simulink model "c960x4096_x14_7_r2013b_frb"  (R2013b)
(part 2 of 79)

      |     t = current_types(ctr);
      |     if (t < 0) || (t > 2),
      |         problem = t;
      |         ctr = numios + 1;
      |     end
      | end
      | if problem ~= 0,
      |     error('Type cannot be %i, must be 0, 1 or 2.', problem);
      | end
      mask Callback bin_pts:
      | swreg_maskcheck(gcb);
      | % blk = gcb;
      | % mode = get_param(blk, 'mode');
      | % current_bins = eval(get_param(blk, 'bin_pts'));
      | % if (strcmp(mode, 'one value') || strcmp(mode, 'fields of equal size')) && (length(current_bins) > 1),
      | %     error('Only one binary pt may be specified for this mode.');
      | % elseif strcmp(mode, 'fields of arbitrary size')
      | %     current_names = textscan(strtrim(strrep(strrep(get_param(blk, 'names'), ']', ''), '[', '')), '%s');
      | %     current_names = current_names{1};
      | %     numios = length(current_names);
      | %     if length(current_bins) ~= numios,
      | %         error('%d field names specified, but %d binary pts?', numios, length(current_bins));
      | %     end
      | % end
  trickler : Subsystem  mask{vec_len_bits=11}
      mask prompts: vec_len_bits "Vector Length (2^?)"
  trig : Subsystem  Tag=xps:sw_reg  AncestorBlock=xps_library/software register  mask(swreg){mode=one value, io_dir=From Processor, io_delay=0, sample_period=1, names=reg, bitwidths=32, arith_types=0, bin_pts=0, sim_port=on, show_format=off}
      mask prompts: io_dir "I/O direction"; io_delay "I/O delay"; sample_period "Sample period"; names "Name:"; bitwidths "Bitwidth:"; arith_types "Type (ufix=0, fix=1, bool=2):"; bin_pts "Binary pt:"; sim_port "Provide sim input/output?"; show_format "Print format string?"
      mask init:
      | swreg_init(gcb)
      settings: AttributesFormatString=1input
      mask TypeOptions mode: one value | fields of equal size | fields of arbitrary size
      mask Callback mode: swreg_cb(gcb);
      mask TypeOptions io_dir: To Processor | From Processor
      mask Callback io_dir:
      | mask_enables = get_param(gcb, 'MaskEnables');
      | mask_names = get_param(gcb, 'MaskNames');
      | if strcmp(get_param(gcb, 'io_dir'), 'To Processor'),
      |     mask_enables{ismember(mask_names, 'sample_period')} = 'off';
      | else
      |     mask_enables{ismember(mask_names, 'sample_period')} = 'on';
      | end
      | set_param(gcb, 'MaskEnables', mask_enables);
      mask Callback bitwidths:
      | swreg_maskcheck(gcb);
      | % blk = gcb;
      | % mode = get_param(blk, 'mode');
      | % current_widths = eval(get_param(blk, 'bitwidths'));
      | % if (strcmp(mode, 'one value') || strcmp(mode, 'fields of equal size')) && (length(current_widths) > 1),
      | %     error('Only one width may be specified for this mode.');
      | % elseif strcmp(mode, 'fields of arbitrary size')
      | %     current_names = textscan(strtrim(strrep(strrep(get_param(blk, 'names'), ']', ''), '[', '')), '%s');
      | %     current_names = current_names{1};
      | %     numios = length(current_names);
      | %     if length(current_widths) ~= numios,
      | %         error('%d field names specified, but %d widths?', numios, length(current_widths));
      | %     end
      | % end
      | % total_width = 0;
      | % for ctr = 1 : length(current_widths),
      | %     total_width = total_width + current_widths(ctr);
      | % end
      | % if total_width > 32,
      | %     error('Total width must be 32 or less, set to %d.', total_width);
      | % end
      mask Callback arith_types:
      | [numios, ~, ~, ~, current_types] = swreg_maskcheck(gcb);
      | % blk = gcb;
      | % mode = get_param(blk, 'mode');
      | % current_types = eval(get_param(blk, 'arith_types'));
      | % numios = length(current_types);
      | % if (strcmp(mode, 'one value') || strcmp(mode, 'fields of equal size')) && (length(current_types) > 1),
      | %     error('Only one type may be specified for this mode.');
      | % elseif strcmp(mode, 'fields of arbitrary size')
      | %     current_names = textscan(strtrim(strrep(strrep(get_param(blk, 'names'), ']', ''), '[', '')), '%s');
      | %     current_names = current_names{1};
      | %     numios = length(current_names);
      | %     if length(current_types) ~= numios,
      | %         error('%d field names specified, but %d types?', numios, length(current_types));
      | %     end
      | % end
      | problem = 0;
      | for ctr = 1 : numios,
      |     t = current_types(ctr);
      |     if (t < 0) || (t > 2),
      |         problem = t;
      |         ctr = numios + 1;
      |     end
      | end
      | if problem ~= 0,
      |     error('Type cannot be %i, must be 0, 1 or 2.', problem);
      | end
      mask Callback bin_pts:
      | swreg_maskcheck(gcb);
      | % blk = gcb;
      | % mode = get_param(blk, 'mode');
      | % current_bins = eval(get_param(blk, 'bin_pts'));
      | % if (strcmp(mode, 'one value') || strcmp(mode, 'fields of equal size')) && (length(current_bins) > 1),
      | %     error('Only one binary pt may be specified for this mode.');
      | % elseif strcmp(mode, 'fields of arbitrary size')
      | %     current_names = textscan(strtrim(strrep(strrep(get_param(blk, 'names'), ']', ''), '[', '')), '%s');
      | %     current_names = current_names{1};
      | %     numios = length(current_names);
      | %     if length(current_bins) ~= numios,
      | %         error('%d field names specified, but %d binary pts?', numios, length(current_bins));
      | %     end
      | % end
  tvg_cmult : Subsystem
  vacc : Subsystem
  wires:
  fftshift/1(in_reg) -> Delay16/1, Delay1/1
  Constant/1 -> fftshift/1(sim_1)
  scale_p0/1(in_reg) -> Delay2/1
  Constant29/1 -> scale_p0/1(sim_1)
  scale_p1/1(in_reg) -> Delay3/1
  Constant2/1 -> scale_p1/1(sim_1)
  ip_1/1(in_reg) -> Delay9/1
  Constant7/1 -> ip_1/1(sim_1)
  ip_2/1(in_reg) -> Delay10/1
  Constant8/1 -> ip_2/1(sim_1)
  ip_3/1(in_reg) -> Delay11/1
  Constant9/1 -> ip_3/1(sim_1)
  ip_4/1(in_reg) -> Delay12/1
  Constant10/1 -> ip_4/1(sim_1)
  ip_5/1(in_reg) -> Delay13/1
  Constant11/1 -> ip_5/1(sim_1)
  ip_6/1(in_reg) -> Delay14/1
  Constant12/1 -> ip_6/1(sim_1)
  ip_7/1(in_reg) -> Delay15/1
  Constant13/1 -> ip_7/1(sim_1)
  Constant15/1 -> pt_1/1(sim_1)
  Constant16/1 -> pt_2/1(sim_1)
  Constant17/1 -> pt_3/1(sim_1)
  Constant18/1 -> pt_4/1(sim_1)
  Constant19/1 -> pt_5/1(sim_1)
  Constant20/1 -> pt_6/1(sim_1)
  Constant21/1 -> pt_7/1(sim_1)
  arm/1(in_reg) -> Slice13/1
  [ADC_SYNC] -> Logical/1
  [P0_FFT_SYNC] -> leds/1(FFT_SYNC)
  [ADC_SYNC] -> leds/2(1PPS)
  Constant5/1 -> n_chan/1(sim_1)
  [TXOF] -> gbe_overflow/1(out_reg)
  Slice2/1 -> Delay4/1
  Register14/1 -> Register13/1
  Register28/1 -> Register27/1
  Register30/1 -> Register29/1
  Constant23/1 -> trig/1(sim_1)
  trig/1(in_reg) -> Slice4/1
  Constant27/1 -> adcsnap0/2(we)
  Constant26/1 -> adcsnap1/2(we)
  [trig] -> adcsnap0/3(trig)
  [trig] -> adcsnap1/3(trig)
  Register49/1 -> Register48/1
  Constant25/1 -> timesel/1(sim_1)
  timesel/1(in_reg) -> Convert16/1
  Convert16/1 -> Delay6/1
  Xilinx14_7/1 -> plat_bd/1(out_reg)
  p0_scale/7(S5_out) -> [P0_S5]
  p0_scale/5(S3_out) -> [P0_S3]
  p0_scale/3(S1_out) -> [P0_S1]
  p0_scale/9(S7_out) -> [P0_S7]
  p0_scale/4(S2_out) -> [P0_S2]
  p0_scale/6(S4_out) -> [P0_S4]
  p0_scale/8(S6_out) -> [P0_S6]
  p0_scale/2(SO_out) -> [P0_S0]
  p1_scale/2(SO_out) -> [P1_S0]
  p1_scale/7(S5_out) -> [P1_S5]
  p1_scale/9(S7_out) -> [P1_S7]
  p1_scale/6(S4_out) -> [P1_S4]
  p1_scale/3(S1_out) -> [P1_S1]
  p1_scale/4(S2_out) -> [P1_S2]
  p1_scale/5(S3_out) -> [P1_S3]
  p1_scale/8(S6_out) -> [P1_S6]
  [P0_S2] -> merge_pol/4(P0_S2)
  [P1_S6] -> merge_pol/16(P1_S6)
  [P0_S5] -> merge_pol/7(P0_S5)
  [P1_S5] -> merge_pol/15(P1_S5)
  [P1_S7] -> merge_pol/17(P1_S7)
  [P0_S4] -> merge_pol/6(P0_S4)
  [P0_S3] -> merge_pol/5(P0_S3)
  [P1_S3] -> merge_pol/13(P1_S3)
  [P1_S1] -> merge_pol/11(P1_S1)
  [P0_S7] -> merge_pol/9(P0_S7)
  [P0_S0] -> merge_pol/2(P0_S0)
  [P0_S1] -> merge_pol/3(P0_S1)
  [P1_S4] -> merge_pol/14(P1_S4)
  [P1_S0] -> merge_pol/10(P1_S0)
  [P0_S6] -> merge_pol/8(P0_S6)
  [P1_S2] -> merge_pol/12(P1_S2)
  [MDB1] -> ds_to_tgbe/2(DIN1)
  [MDB2] -> ds_to_tgbe/3(DIN2)
  [MDB3] -> ds_to_tgbe/4(DIN3)
  [MSYNC1] -> ds_to_tgbe/5(MSYNC)
  [SYNC] -> ds_to_tgbe/6(SYNCIN)
  [NCHAN] -> ds_to_tgbe/7(NCHAN)
  ds_to_tgbe/11(STB_3) -> [STB_3]
  ds_to_tgbe/19(DOUT_6) -> [DOUT_6]
  ds_to_tgbe/21(EOF_6) -> [EOF_6]
  ds_to_tgbe/18(EOF_5) -> [EOF_5]
  ds_to_tgbe/24(EOF_7) -> [EOF_7]
  ds_to_tgbe/22(DOUT_7) -> [DOUT_7]
  ds_to_tgbe/5(STB_1) -> [STB_1]
  ds_to_tgbe/17(STB_5) -> [STB_5]
  ds_to_tgbe/16(DOUT_5) -> [DOUT_5]
  ds_to_tgbe/3(EOF_0) -> [EOF_0]
  ds_to_tgbe/15(EOF_4) -> [EOF_4]
  ds_to_tgbe/14(STB_4) -> [STB_4]
  ds_to_tgbe/9(EOF_2) -> [EOF_2]
  ds_to_tgbe/10(DOUT_3) -> [DOUT_3]
  ds_to_tgbe/20(STB_6) -> [STB_6]
  ds_to_tgbe/23(STB_7) -> [STB_7]
  ds_to_tgbe/2(STB_0) -> [STB_0]
  ds_to_tgbe/12(EOF_3) -> [EOF_3]
  ds_to_tgbe/4(DOUT_1) -> [DOUT_1]
  ds_to_tgbe/7(DOUT_2) -> [DOUT_2]
  ds_to_tgbe/6(EOF_1) -> [EOF_1]
  ds_to_tgbe/8(STB_2) -> [STB_2]
  ds_to_tgbe/13(DOUT_4) -> [DOUT_4]
  RUNT_7/2(EOF_OUT) -> [REOF_7]
  RUNT_7/1(STB_OUT) -> [RSTB_7]
  [EOF_7] -> RUNT_7/3(EOF)
  [STB_7] -> RUNT_7/2(STB)
  [MSYNC2] -> RUNT_7/1(MSYNC)
  RUNT_6/2(EOF_OUT) -> [REOF_6]
  RUNT_6/1(STB_OUT) -> [RSTB_6]
  [EOF_6] -> RUNT_6/3(EOF)
  [STB_6] -> RUNT_6/2(STB)
  [MSYNC2] -> RUNT_6/1(MSYNC)
  RUNT_5/2(EOF_OUT) -> [REOF_5]
  RUNT_5/1(STB_OUT) -> [RSTB_5]
  [EOF_5] -> RUNT_5/3(EOF)
  [STB_5] -> RUNT_5/2(STB)
  [MSYNC2] -> RUNT_5/1(MSYNC)
  RUNT_4/2(EOF_OUT) -> [REOF_4]
  RUNT_4/1(STB_OUT) -> [RSTB_4]
  [EOF_4] -> RUNT_4/3(EOF)
  [STB_4] -> RUNT_4/2(STB)
  [MSYNC2] -> RUNT_4/1(MSYNC)
  RUNT_3/2(EOF_OUT) -> [REOF_3]
  RUNT_3/1(STB_OUT) -> [RSTB_3]
  [EOF_3] -> RUNT_3/3(EOF)
  [STB_3] -> RUNT_3/2(STB)
  [MSYNC2] -> RUNT_3/1(MSYNC)
  RUNT_2/2(EOF_OUT) -> [REOF_2]
  RUNT_2/1(STB_OUT) -> [RSTB_2]
  [EOF_2] -> RUNT_2/3(EOF)
  [STB_2] -> RUNT_2/2(STB)
  [MSYNC2] -> RUNT_2/1(MSYNC)
  RUNT_1/2(EOF_OUT) -> [REOF_1]
  RUNT_1/1(STB_OUT) -> [RSTB_1]
  [EOF_1] -> RUNT_1/3(EOF)
  [STB_1] -> RUNT_1/2(STB)
  [MSYNC2] -> RUNT_1/1(MSYNC)
  RUNT_0/2(EOF_OUT) -> [REOF_0]
  RUNT_0/1(STB_OUT) -> [RSTB_0]
  [EOF_0] -> RUNT_0/3(EOF)
  [STB_0] -> RUNT_0/2(STB)
  [MSYNC2] -> RUNT_0/1(MSYNC)
  Constant34/1 -> Concat/1
  [TXOF_7] -> Concat/2
  [TXOF_6] -> Concat/3
  [TXOF_5] -> Concat/4
  [TXOF_4] -> Concat/5
  [TXOF_3] -> Concat/6
  [TXOF_2] -> Concat/7
  [TXOF_1] -> Concat/8
  [TXOF_0] -> Concat/9
  [RESET_7] -> gbe7/1
  Constant33/1 -> gbe7/8
  Constant32/1 -> gbe7/7
  gbe7/12 -> Terminator81/1
  gbe7/11 -> Terminator80/1
  gbe7/10 -> Terminator90/1
  gbe7/9 -> Terminator89/1
  gbe7/8 -> Terminator88/1
  gbe7/7 -> Terminator87/1
  gbe7/6 -> Terminator86/1
  gbe7/5 -> [TXOF_7]
  gbe7/4 -> Terminator84/1
  gbe7/3 -> Terminator83/1
  gbe7/2 -> Terminator79/1
  gbe7/1 -> Terminator78/1
  [RESET_6] -> gbe6/1
  Constant31/1 -> gbe6/8
  Constant30/1 -> gbe6/7
  gbe6/12 -> Terminator68/1
  gbe6/11 -> Terminator67/1
  gbe6/10 -> Terminator77/1
  gbe6/9 -> Terminator76/1
  gbe6/8 -> Terminator75/1
  gbe6/7 -> Terminator74/1
  gbe6/6 -> Terminator73/1
  gbe6/5 -> [TXOF_6]
  gbe6/4 -> Terminator70/1
  gbe6/3 -> Terminator69/1
  gbe6/2 -> Terminator66/1
  gbe6/1 -> Terminator65/1
  [RESET_5] -> gbe5/1
  Constant28/1 -> gbe5/8
  Constant4/1 -> gbe5/7
  gbe5/12 -> Terminator55/1
  gbe5/11 -> Terminator54/1
  gbe5/10 -> Terminator64/1
  gbe5/9 -> Terminator63/1
  gbe5/8 -> Terminator62/1
  gbe5/7 -> Terminator61/1
  gbe5/6 -> Terminator59/1
  gbe5/5 -> [TXOF_5]
  gbe5/4 -> Terminator57/1
  gbe5/3 -> Terminator56/1
  gbe5/2 -> Terminator53/1
  gbe5/1 -> Terminator52/1
  [RESET_4] -> gbe4/1
  Constant42/1 -> gbe4/8
  Constant41/1 -> gbe4/7
  gbe4/12 -> Terminator51/1
  gbe4/11 -> Terminator50/1
  gbe4/10 -> Terminator95/1
  gbe4/9 -> Terminator94/1
  gbe4/8 -> Terminator93/1
  gbe4/7 -> Terminator92/1
  gbe4/6 -> Terminator91/1
  gbe4/5 -> [TXOF_4]
  gbe4/4 -> Terminator71/1
  gbe4/3 -> Terminator60/1
  gbe4/2 -> Terminator49/1
  gbe4/1 -> Terminator48/1
  Constant40/1 -> gbe3/8
  Constant39/1 -> gbe3/7
  gbe3/12 -> Terminator39/1
  gbe3/11 -> Terminator38/1
  gbe3/10 -> Terminator47/1
  gbe3/9 -> Terminator46/1
  gbe3/8 -> Terminator45/1
  gbe3/7 -> Terminator44/1
  gbe3/6 -> Terminator6/1
  gbe3/5 -> [TXOF_3]
  gbe3/4 -> Terminator41/1
  gbe3/3 -> Terminator40/1
  gbe3/2 -> Terminator37/1
  gbe3/1 -> Terminator36/1
  Constant38/1 -> gbe2/8
  Constant37/1 -> gbe2/7
  gbe2/12 -> Terminator27/1
  gbe2/11 -> Terminator26/1
  gbe2/10 -> Terminator35/1
  gbe2/9 -> Terminator34/1
  gbe2/8 -> Terminator33/1
  gbe2/7 -> Terminator32/1
  gbe2/6 -> Terminator31/1
  gbe2/5 -> [TXOF_2]
  gbe2/4 -> Terminator29/1
  gbe2/3 -> Terminator28/1
  gbe2/2 -> Terminator25/1
  gbe2/1 -> Terminator24/1
  Constant36/1 -> gbe1/8
  Constant35/1 -> gbe1/7
  gbe1/12 -> Terminator15/1
  gbe1/11 -> Terminator14/1
  gbe1/10 -> Terminator23/1
  gbe1/9 -> Terminator22/1
  gbe1/8 -> Terminator21/1
  gbe1/7 -> Terminator20/1
  gbe1/6 -> Terminator19/1
  gbe1/5 -> [TXOF_1]
  gbe1/4 -> Terminator17/1
  gbe1/3 -> Terminator16/1
  gbe1/2 -> Terminator13/1
  [REOF_0] -> gbe0/6
  [PT_0] -> gbe0/5
  [IP_0] -> gbe0/4
  [RSTB_0] -> gbe0/3
  [DOUT_0] -> gbe0/2
  Constant3/1 -> gbe0/8
  Constant1/1 -> gbe0/7
  gbe0/12 -> Terminator11/1
  gbe0/11 -> Terminator10/1
  gbe0/10 -> Terminator42/1
  gbe0/9 -> Terminator30/1
  gbe0/8 -> Terminator18/1
  gbe0/7 -> Terminator9/1
  gbe0/6 -> Terminator7/1
  gbe0/5 -> [TXOF_0]
  gbe0/4 -> Terminator5/1
  gbe0/3 -> Terminator4/1
  gbe0/2 -> Terminator2/1
  [REOF_7] -> gbe7/6
  [PT_7] -> gbe7/5
  [IP_7] -> gbe7/4
  [RSTB_7] -> gbe7/3
  [DOUT_7] -> gbe7/2
  [REOF_6] -> gbe6/6
  [PT_6] -> gbe6/5
  [IP_6] -> gbe6/4
  [RSTB_6] -> gbe6/3
  [DOUT_6] -> gbe6/2
  [REOF_5] -> gbe5/6
  [PT_5] -> gbe5/5
  [IP_5] -> gbe5/4
  [RSTB_5] -> gbe5/3
  [DOUT_5] -> gbe5/2
  [REOF_4] -> gbe4/6
  [PT_4] -> gbe4/5
  [IP_4] -> gbe4/4
  [RSTB_4] -> gbe4/3
  [DOUT_4] -> gbe4/2
  [REOF_3] -> gbe3/6
  [PT_3] -> gbe3/5
  [IP_3] -> gbe3/4
  [RSTB_3] -> gbe3/3
  [DOUT_3] -> gbe3/2
  [RESET_3] -> gbe3/1
  [REOF_2] -> gbe2/6
  [PT_2] -> gbe2/5
  [IP_2] -> gbe2/4
  [RSTB_2] -> gbe2/3
  [DOUT_2] -> gbe2/2
  [RESET_2] -> gbe2/1
  [REOF_1] -> gbe1/6
  [PT_1] -> gbe1/5
  [IP_1] -> gbe1/4
  [RSTB_1] -> gbe1/3
  [DOUT_1] -> gbe1/2
  [spec_tick] -> ssg/2(spec_tick)
  AddSub/1 -> Convert/1
  Convert/1 -> Register1/1
  Constant43/1 -> AddSub/2
  [N_CHAN] -> AddSub/1
  [ARM] -> arm_ss/1(ARM_INPUT)
  arm_ss/1(MSYNC_OUT) -> [MSYNC]
  [P0_ADC] -> adcsnap0/1(din)
  [P1_ADC] -> adcsnap1/1(din)
  [MSYNC] -> Register44/1
  Register44/1 -> Register7/1
  Register8/1 -> Register12/1
  Register12/1 -> [MSYNC0]
  Register48/1 -> [MSYNC1]
  Register13/1 -> [MSYNC2]
  Register27/1 -> [MSYNC3]
  Register29/1 -> [MSYNC4]
  Register7/1 -> Register28/1, Register30/1, Register49/1, Register8/1, Register14/1
  c1500x4096_ss/1 -> design_id/1(out_reg)
  Slice4/1 -> edge_detect2/1(in)
  edge_detect2/1(out) -> Delay5/1
  n_chan/1(in_reg) -> Slice2/1
  Slice13/1 -> edge_detect4/1(in)
  Constant22/1 -> arm/1(sim_1)
  Delay1/1 -> [FFT_SHIFT_0]
  Delay2/1 -> [SCALE_P0]
  Delay3/1 -> [SCALE_P1]
  Delay4/1 -> [N_CHAN]
  Delay5/1 -> [trig]
  Delay6/1 -> [timesel]
  edge_detect4/1(out) -> Delay/1
  Delay/1 -> [ARM]
  Constant6/1 -> ip_0/1(sim_1)
  ip_0/1(in_reg) -> Delay8/1
  Delay8/1 -> [IP_0]
  Delay9/1 -> [IP_1]
  Delay10/1 -> [IP_2]
  Delay11/1 -> [IP_3]
  Delay12/1 -> [IP_4]
  Delay13/1 -> [IP_5]
  Delay14/1 -> [IP_6]
  Delay15/1 -> [IP_7]
  Delay16/1 -> [FFT_SHIFT_1]
  Constant14/1 -> pt_0/1(sim_1)
  pt_0/1(in_reg) -> Delay17/1
  Delay17/1 -> [PT_0]
  pt_1/1(in_reg) -> Delay18/1
  pt_2/1(in_reg) -> Delay19/1
  pt_3/1(in_reg) -> Delay20/1
  pt_4/1(in_reg) -> Delay21/1
  pt_5/1(in_reg) -> Delay22/1
  pt_6/1(in_reg) -> Delay23/1
  pt_7/1(in_reg) -> Delay24/1
  Delay18/1 -> [PT_1]
  Delay19/1 -> [PT_2]
  Delay20/1 -> [PT_3]
  Delay21/1 -> [PT_4]
  Delay22/1 -> [PT_5]
  Delay23/1 -> [PT_6]
  Delay24/1 -> [PT_7]
  Register58/1 -> ssg/1(reset)
  [MSYNC4] -> Register58/1
  Constant24/1 -> reset/1(sim_1)
  [MSYNC3] -> spec_tick_gen/1(In)
  spec_tick_gen/1(Out) -> [spec_tick]
  Delay27/1 -> p0_scale/1(sync)
  Delay28/1 -> p0_scale/2(S0)
  Delay29/1 -> p0_scale/3(S1)
  Delay30/1 -> p0_scale/4(S2)
  Delay31/1 -> p0_scale/5(S3)
  Delay32/1 -> p0_scale/6(S4)
  Delay33/1 -> p0_scale/7(S5)
  Delay34/1 -> p0_scale/8(S6)
  Delay35/1 -> p0_scale/9(S7)
  Delay36/1 -> p1_scale/1(sync)
  Delay37/1 -> p1_scale/2(S0)
  Delay38/1 -> p1_scale/3(S1)
  Delay39/1 -> p1_scale/4(S2)
  Delay40/1 -> p1_scale/5(S3)
  Delay41/1 -> p1_scale/6(S4)
  Delay42/1 -> p1_scale/7(S5)
  Delay43/1 -> p1_scale/8(S6)
  Delay44/1 -> p1_scale/9(S7)
  p0_scale/1(sync_out) -> [P0_FFT_SYNC]
  p1_scale/1(sync_out) -> 05_OCT_4/1
  [P0_FFT_SYNC] -> merge_pol/1(sync)
  merge_pol/1(sync_out) -> Delay45/1
  Delay45/1 -> [SYNC]
  merge_pol/2(MDB0) -> Delay46/1
  Delay46/1 -> [MDB0]
  merge_pol/3(MDB1) -> Delay47/1
  Delay47/1 -> [MDB1]
  merge_pol/4(MDB2) -> Delay48/1
  Delay48/1 -> [MDB2]
  merge_pol/5(MDB3) -> Delay49/1
  Delay49/1 -> [MDB3]
  [MDB0] -> ds_to_tgbe/1(DIN0)
  ds_to_tgbe/1(DOUT_0) -> [DOUT_0]
  [RESET_0] -> gbe0/1
  [RESET_1] -> gbe1/1
  gbe1/1 -> Terminator3/1
  Concat/1 -> [TXOF]
  [SCALE_P0] -> p0_scale/10(SCALE)
  [SCALE_P1] -> p1_scale/10(SCALE)
  reset/1(in_reg) -> RUNT_RESET_LOGIC/1(In1)
  RUNT_RESET_LOGIC/1(Out1) -> [RESET_0]
  RUNT_RESET_LOGIC/2(Out2) -> [RESET_1]
  RUNT_RESET_LOGIC/3(Out3) -> [RESET_2]
  RUNT_RESET_LOGIC/4(Out4) -> [RESET_3]
  RUNT_RESET_LOGIC/5(Out5) -> [RESET_4]
  RUNT_RESET_LOGIC/6(Out6) -> [RESET_5]
  RUNT_RESET_LOGIC/7(Out7) -> [RESET_6]
  RUNT_RESET_LOGIC/8(Out8) -> [RESET_7]
  design_id/1(sim_out) -> 16_DEC_15/1
  plat_bd/1(sim_out) -> 16_DEC_15_01/1
  gbe_overflow/1(sim_out) -> 05_OCT_15_02/1
  Register1/1 -> [NCHAN]
  [F0_S0] -> Delay26/1
  [F0_S1] -> Delay50/1
  [F0_S2] -> Delay51/1
  [F0_S3] -> Delay52/1
  [F0_S4] -> Delay53/1
  [F0_S5] -> Delay54/1
  [F0_S6] -> Delay55/1
  [F1_S5] -> Delay62/1
  [F1_S7] -> Delay64/1
  [F1_S4] -> Delay61/1
  [F1_S0] -> Delay57/1
  [F1_S3] -> Delay60/1
  [F1_S6] -> Delay63/1
  [F1_S1] -> Delay58/1
  [F1_S2] -> Delay59/1
  [F0_S7] -> Delay56/1
  cross_corr/2(xx*) -> tvg_cmult/2(xx)
  cross_corr/3(xy*) -> tvg_cmult/3(xy)
  cross_corr/4(yy*) -> tvg_cmult/4(yy)
  rst_cpoge/1(in_reg) -> Slice1/1
  Slice1/1 -> [rst]
  Constant44/1 -> rst_cpoge/1(sim_1)
  p0_adc/1(P0_DS) -> [P0_ADC], bus_expand/1(bus_in)
  p0_adc/2(1PPS) -> [ADC_SYNC]
  p1_adc/1(P0_DS) -> [P1_ADC], bus_expand2/1(bus_in)
  p1_adc/2(1PPS) -> 05_OCT_1/1
  codd_fft_4096ch_p1/2 -> [F1_S0]
  codd_fft_4096ch_p1/3 -> [F1_S1]
  codd_fft_4096ch_p1/4 -> [F1_S2]
  codd_fft_4096ch_p1/5 -> [F1_S3]
  codd_fft_4096ch_p1/6 -> [F1_S4]
  codd_fft_4096ch_p1/7 -> [F1_S5]
  codd_fft_4096ch_p1/8 -> [F1_S6]
  codd_fft_4096ch_p1/9 -> [F1_S7]
  bus_expand/2(out15) -> [P0_1]
  bus_expand/3(out14) -> [P0_2]
  bus_expand/4(out13) -> [P0_3]
  bus_expand/5(out12) -> [P0_4]
  bus_expand/6(out11) -> [P0_5]
  bus_expand/7(out10) -> [P0_6]
  bus_expand/16(lsb_out1) -> [P0_15]
  bus_expand/12(out5) -> [P0_11]
  bus_expand/13(out4) -> [P0_12]
  bus_expand/14(out3) -> [P0_13]
  bus_expand/15(out2) -> [P0_14]
  bus_expand/8(out9) -> [P0_7]
  bus_expand/9(out8) -> [P0_8]
  bus_expand/10(out7) -> [P0_9]
  bus_expand/11(out6) -> [P0_10]
  bus_expand2/1(msb_out16) -> [P1_0]
  bus_expand2/2(out15) -> [P1_1]
  bus_expand2/15(out2) -> [P1_14]
  bus_expand2/16(lsb_out1) -> [P1_15]
  bus_expand2/11(out6) -> [P1_10]
  bus_expand2/12(out5) -> [P1_11]
  bus_expand2/13(out4) -> [P1_12]
  bus_expand2/14(out3) -> [P1_13]
  bus_expand2/7(out10) -> [P1_6]
  bus_expand2/8(out9) -> [P1_7]
  bus_expand2/9(out8) -> [P1_8]
  bus_expand2/10(out7) -> [P1_9]
  bus_expand2/3(out14) -> [P1_2]
  bus_expand2/4(out13) -> [P1_3]
  bus_expand2/5(out12) -> [P1_4]
  bus_expand2/6(out11) -> [P1_5]
  bus_expand/1(msb_out16) -> [P0_0]
  [P1_15] -> codd_pfb_4096ch/33
  codd_fft_4096ch_p1/10 -> 05_OCT_3/1
  [MSYNC0] -> codd_pfb_4096ch/1
  [P0_0] -> codd_pfb_4096ch/2
  [P1_0] -> codd_pfb_4096ch/3
  [P0_1] -> codd_pfb_4096ch/4
  [P1_1] -> codd_pfb_4096ch/5
  [P0_2] -> codd_pfb_4096ch/6
  [P1_2] -> codd_pfb_4096ch/7
  [P0_3] -> codd_pfb_4096ch/8
  [P1_3] -> codd_pfb_4096ch/9
  [P0_4] -> codd_pfb_4096ch/10
  [P1_4] -> codd_pfb_4096ch/11
  [P0_5] -> codd_pfb_4096ch/12
  [P1_5] -> codd_pfb_4096ch/13
  [P0_6] -> codd_pfb_4096ch/14
  [P1_6] -> codd_pfb_4096ch/15
  [P0_7] -> codd_pfb_4096ch/16
  [P1_7] -> codd_pfb_4096ch/17
  [P0_8] -> codd_pfb_4096ch/18
  [P1_8] -> codd_pfb_4096ch/19
  [P0_9] -> codd_pfb_4096ch/20
  [P1_9] -> codd_pfb_4096ch/21
  [P0_10] -> codd_pfb_4096ch/22
  [P1_10] -> codd_pfb_4096ch/23
  [P0_11] -> codd_pfb_4096ch/24
  [P1_11] -> codd_pfb_4096ch/25
  [P0_12] -> codd_pfb_4096ch/26
  [P1_12] -> codd_pfb_4096ch/27
  [P0_13] -> codd_pfb_4096ch/28
  [P1_13] -> codd_pfb_4096ch/29
  [P0_14] -> codd_pfb_4096ch/30
  [P1_14] -> codd_pfb_4096ch/31
  [P0_15] -> codd_pfb_4096ch/32
  codd_pfb_4096ch/33 -> [P1_15_pfbout]
  codd_pfb_4096ch/1 -> [PFB_SYNC]
  codd_pfb_4096ch/2 -> [P0_0_pfbout]
  codd_pfb_4096ch/3 -> [P1_0_pfbout]
  codd_pfb_4096ch/4 -> [P0_1_pfbout]
  codd_pfb_4096ch/5 -> [P1_1_pfbout]
  codd_pfb_4096ch/6 -> [P0_2_pfbout]
  codd_pfb_4096ch/7 -> [P1_2_pfbout]
  codd_pfb_4096ch/8 -> [P0_3_pfbout]
  codd_pfb_4096ch/9 -> [P1_3_pfbout]
  codd_pfb_4096ch/10 -> [P0_4_pfbout]
  codd_pfb_4096ch/11 -> [P1_4_pfbout]
  codd_pfb_4096ch/12 -> [P0_5_pfbout]
  codd_pfb_4096ch/13 -> [P1_5_pfbout]
  codd_pfb_4096ch/14 -> [P0_6_pfbout]
  codd_pfb_4096ch/15 -> [P1_6_pfbout]
  codd_pfb_4096ch/16 -> [P0_7_pfbout]
  codd_pfb_4096ch/17 -> [P1_7_pfbout]
  codd_pfb_4096ch/18 -> [P0_8_pfbout]
  codd_pfb_4096ch/19 -> [P1_8_pfbout]
  codd_pfb_4096ch/20 -> [P0_9_pfbout]
  codd_pfb_4096ch/21 -> [P1_9_pfbout]
  codd_pfb_4096ch/22 -> [P0_10_pfbout]
  codd_pfb_4096ch/23 -> [P1_10_pfbout]
  codd_pfb_4096ch/24 -> [P0_11_pfbout]
  codd_pfb_4096ch/25 -> [P1_11_pfbout]
  codd_pfb_4096ch/26 -> [P0_12_pfbout]
  codd_pfb_4096ch/27 -> [P1_12_pfbout]
  codd_pfb_4096ch/28 -> [P0_13_pfbout]
  codd_pfb_4096ch/29 -> [P1_13_pfbout]
  codd_pfb_4096ch/30 -> [P0_14_pfbout]
  codd_pfb_4096ch/31 -> [P1_14_pfbout]
  codd_pfb_4096ch/32 -> [P0_15_pfbout]
  codd_fft_4096ch_p0/3 -> [F0_S1]
  codd_fft_4096ch_p0/4 -> [F0_S2]
  codd_fft_4096ch_p0/5 -> [F0_S3]
  codd_fft_4096ch_p0/6 -> [F0_S4]
  codd_fft_4096ch_p0/7 -> [F0_S5]
  codd_fft_4096ch_p0/8 -> [F0_S6]
  codd_fft_4096ch_p0/9 -> [F0_S7]
  codd_fft_4096ch_p0/10 -> 05_OCT_2/1
  codd_fft_4096ch_p0/2 -> [F0_S0]
  [FFT_SHIFT_1] -> codd_fft_4096ch_p1/2
  [PFB_SYNC] -> codd_fft_4096ch_p1/1
  [P1_7_pfbout] -> codd_fft_4096ch_p1/10
  [P1_8_pfbout] -> codd_fft_4096ch_p1/11
  [P1_4_pfbout] -> codd_fft_4096ch_p1/7
  [P1_9_pfbout] -> codd_fft_4096ch_p1/12
  [P1_10_pfbout] -> codd_fft_4096ch_p1/13
  [P1_15_pfbout] -> codd_fft_4096ch_p1/18
  [P1_11_pfbout] -> codd_fft_4096ch_p1/14
  [P1_12_pfbout] -> codd_fft_4096ch_p1/15
  [P1_5_pfbout] -> codd_fft_4096ch_p1/8
  [P1_6_pfbout] -> codd_fft_4096ch_p1/9
  [P1_2_pfbout] -> codd_fft_4096ch_p1/5
  [P1_3_pfbout] -> codd_fft_4096ch_p1/6
  [P1_0_pfbout] -> codd_fft_4096ch_p1/3
  [P1_1_pfbout] -> codd_fft_4096ch_p1/4
  [P1_13_pfbout] -> codd_fft_4096ch_p1/16
  [P1_14_pfbout] -> codd_fft_4096ch_p1/17
  [P0_14_pfbout] -> codd_fft_4096ch_p0/17
  [P0_15_pfbout] -> codd_fft_4096ch_p0/18
  [PFB_SYNC] -> codd_fft_4096ch_p0/1
  [FFT_SHIFT_0] -> codd_fft_4096ch_p0/2
  [P0_0_pfbout] -> codd_fft_4096ch_p0/3
  [P0_1_pfbout] -> codd_fft_4096ch_p0/4
  [P0_2_pfbout] -> codd_fft_4096ch_p0/5
  [P0_3_pfbout] -> codd_fft_4096ch_p0/6
  [P0_4_pfbout] -> codd_fft_4096ch_p0/7
  [P0_5_pfbout] -> codd_fft_4096ch_p0/8
  [P0_6_pfbout] -> codd_fft_4096ch_p0/9
  [P0_7_pfbout] -> codd_fft_4096ch_p0/10
  [P0_8_pfbout] -> codd_fft_4096ch_p0/11
  [P0_9_pfbout] -> codd_fft_4096ch_p0/12
  [P0_10_pfbout] -> codd_fft_4096ch_p0/13
  [P0_11_pfbout] -> codd_fft_4096ch_p0/14
  [P0_12_pfbout] -> codd_fft_4096ch_p0/15
  [P0_13_pfbout] -> codd_fft_4096ch_p0/16
  codd_fft_4096ch_p0/1 -> [F0_FFT_SYNC]
  codd_fft_4096ch_p1/1 -> [F1_FFT_SYNC]
  [F0_FFT_SYNC] -> Delay27/1
  [F0_S0] -> Delay28/1
  [F0_S1] -> Delay29/1
  [F0_S2] -> Delay30/1
  [F0_S3] -> Delay31/1
  [F0_S4] -> Delay32/1
  [F0_S5] -> Delay33/1
  [F0_S6] -> Delay34/1
  [F0_S7] -> Delay35/1
  [F1_FFT_SYNC] -> Delay36/1
  [F1_S0] -> Delay37/1
  [F1_S1] -> Delay38/1
  [F1_S2] -> Delay39/1
  [F1_S3] -> Delay40/1
  [F1_S4] -> Delay41/1
  [F1_S5] -> Delay42/1
  [F1_S6] -> Delay43/1
  [F1_S7] -> Delay44/1
  [F0_FFT_SYNC] -> Delay25/1
  tvg_cmult/2(dout0) -> vacc/3(dinxx)
  tvg_cmult/3(dout1) -> vacc/4(dinxy)
  tvg_cmult/4(dout2) -> vacc/5(dinyy)
  tvg_cmult/1(sync_out) -> vacc/2(sync)
  vacc/2(dout) -> trickler/2(din)
  vacc/1(new_acc_out) -> trickler/1(new_acc)
  trickler/1(new_acc_out) -> Packetizer/1(new_acc)
  trickler/3(dout_vld) -> Packetizer/3(din_vld)
  Packetizer/1(dout) -> one_GbE/1(din)
  Packetizer/3(eof) -> one_GbE/3(eof)
  [rst] -> Packetizer/4(rst)
  [rst] -> one_GbE/4(rst)
  [rst] -> vacc/1(rst)
  Packetizer/2(dout_vld) -> one_GbE/2(vld)
  trickler/2(dout) -> Packetizer/2(din)
  cross_corr/1(sync_out) -> tvg_cmult/1(sync)
  sw_pps/1(in_reg) -> Slice3/1
  Slice3/1 -> Delay7/1
  Constant45/1 -> sw_pps/1(sim_1)
  Delay7/1 -> [SW_PPS]
  Logical/1 -> arm_ss/2(1PPS_INPUT)
  [SW_PPS] -> Logical/2
  Delay25/1 -> cross_corr/1(sync)
  Delay26/1 -> cross_corr/2(P0_S0)
  Delay50/1 -> cross_corr/3(P0_S1)
  Delay51/1 -> cross_corr/4(P0_S2)
  Delay52/1 -> cross_corr/5(P0_S3)
  Delay53/1 -> cross_corr/6(P0_S4)
  Delay54/1 -> cross_corr/7(P0_S5)
  Delay55/1 -> cross_corr/8(P0_S6)
  Delay56/1 -> cross_corr/9(P0_S7)
  Delay57/1 -> cross_corr/10(P1_S0)
  Delay58/1 -> cross_corr/11(P1_S1)
  Delay59/1 -> cross_corr/12(P1_S2)
  Delay60/1 -> cross_corr/13(P1_S3)
  Delay61/1 -> cross_corr/14(P1_S4)
  Delay62/1 -> cross_corr/15(P1_S5)
  Delay63/1 -> cross_corr/16(P1_S6)
  Delay64/1 -> cross_corr/17(P1_S7)
